simulink model "microMouseSimulator"  (R2019b)
settings: Solver=FixedStepAuto  StartTime=0.0  StopTime=5  FixedStep=0.1  MinStep=0.1  RelTol=1e-3
undefined symbols (not defined in the file): Rl, Rr, W
settings Model: Creator=r720r  LastModifiedBy=r720r

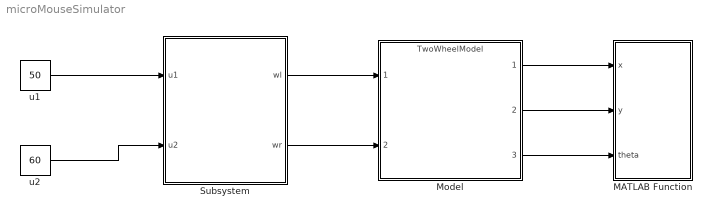
== system microMouseSimulator ==
  MATLAB Function : MATLAB Function  TreatAsAtomicUnit=on
  Model : ModelReference  ModelNameDialog=TwoWheelModel.slx  ModelReferenceVersion=1.3
  Subsystem : Subsystem  TreatAsAtomicUnit=on
  u1 : Constant  Value=50
  u2 : Constant  Value=60
  wires:
  Model/1 -> MATLAB Function/1(x)
  Model/2 -> MATLAB Function/2(y)
  Model/3 -> MATLAB Function/3(theta)
  u1/1 -> Subsystem/1(u1)
  u2/1 -> Subsystem/2(u2)
  Subsystem/1(wl) -> Model/1
  Subsystem/2(wr) -> Model/2

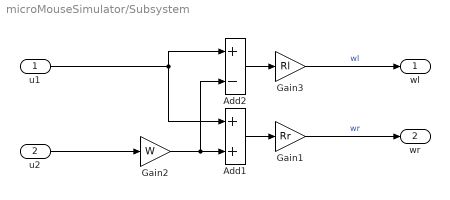
== system microMouseSimulator/Subsystem ==
  u1 : Inport
  u2 : Inport  Port=2
  Add1 : Sum
  Add2 : Sum  Inputs=+-
  Gain1 : Gain  Gain=Rr
  Gain2 : Gain  Gain=W
  Gain3 : Gain  Gain=Rl
  wl : Outport
  wr : Outport  Port=2
  wires:
  Add1/1 -> Gain1/1
  u2/1 -> Gain2/1
  Gain2/1 -> Add2/2, Add1/2
  u1/1 -> Add2/1, Add1/1
  Add2/1 -> Gain3/1
  Gain1/1 -> wr/1  "wr"
  Gain3/1 -> wl/1  "wl"

== matlab function microMouseSimulator/MATLAB Function ==
  data: x input; y input; theta input
function fcn(x, y, theta)
    coder.extrinsic('evalin', 'plot', 'setfield', 'redraw');
    TwoWheel = evalin('base','TwoWheel'); 
    fig = evalin('base','fig'); %ベースワークスペースのハンドル取得
    
    theta_deg = theta * 180 /pi;
    TwoWheel = setfield(TwoWheel, 'X', x);
    TwoWheel = setfield(TwoWheel, 'Y', y);
    TwoWheel = setfield(TwoWheel, 'Theta_deg', theta_deg);
    
    redraw(TwoWheel);
    %set はグラフィックス オブジェクトのプロパティの設定
